simulink model "SCF"  (R2021b)
settings: configuration reference "CommonModelConfiguration" (kept outside this file)
settings Model: Creator=JELIASS5  LastModifiedBy=JELIASS5
settings ConfigSetRef: SourceName=CommonModelConfiguration  SourceLocation=Base Workspace

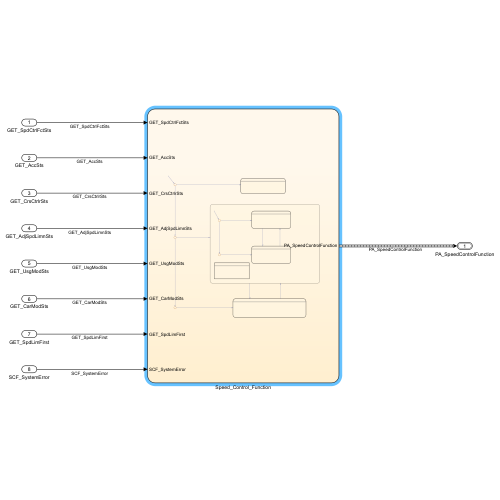
[thumbnail: Simulink's stored preview of the top-level diagram]
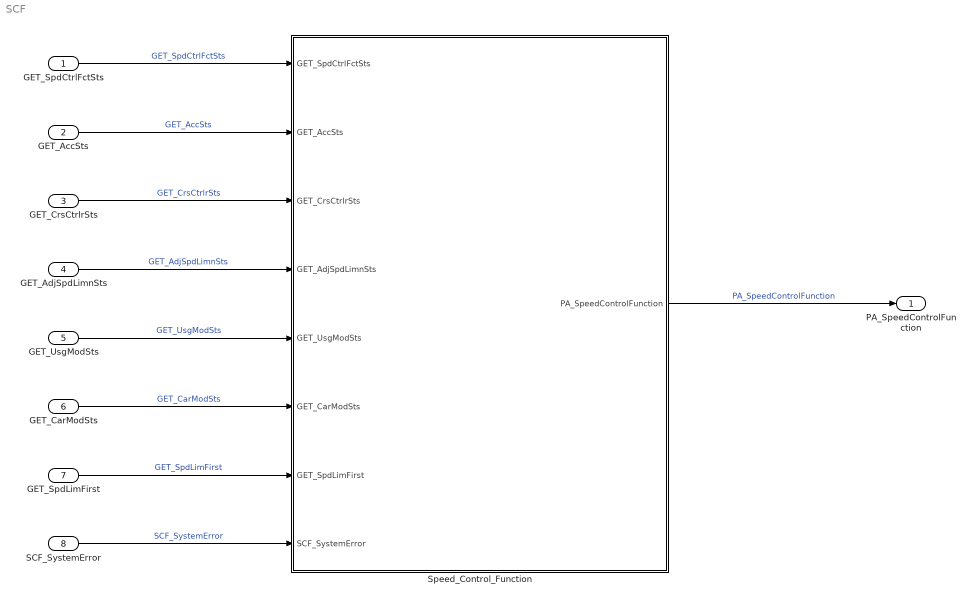
== system SCF ==
  GET_SpdCtrlFctSts : Inport  OutDataTypeStr=Enum: FctStsSpdCtrl
  GET_AccSts : Inport  Port=2  OutDataTypeStr=Enum: AccSts1
  GET_CrsCtrlrSts : Inport  Port=3  OutDataTypeStr=Enum: CrsCtrlrSts1
  GET_AdjSpdLimnSts : Inport  Port=4  OutDataTypeStr=Enum: AdjSpdLimnSts2
  GET_UsgModSts : Inport  Port=5  OutDataTypeStr=Enum: UsgModSts1
  GET_CarModSts : Inport  Port=6  OutDataTypeStr=Enum: CarModSts1
  GET_SpdLimFirst : Inport  Port=7  OutDataTypeStr=SpdLimVal1
  SCF_SystemError : Inport  Port=8  OutDataTypeStr=boolean
  Speed_Control_Function : Stateflow chart  TreatAsAtomicUnit=on
  PA_SpeedControlFunction : Outport  OutDataTypeStr=Bus: PA_StatusAnduIntAndOffOnValue
  wires:
  GET_SpdCtrlFctSts/1 -> Speed_Control_Function/1(GET_SpdCtrlFctSts)  "GET_SpdCtrlFctSts"
  GET_AccSts/1 -> Speed_Control_Function/2(GET_AccSts)  "GET_AccSts"
  GET_CrsCtrlrSts/1 -> Speed_Control_Function/3(GET_CrsCtrlrSts)  "GET_CrsCtrlrSts"
  GET_AdjSpdLimnSts/1 -> Speed_Control_Function/4(GET_AdjSpdLimnSts)  "GET_AdjSpdLimnSts"
  GET_UsgModSts/1 -> Speed_Control_Function/5(GET_UsgModSts)  "GET_UsgModSts"
  GET_CarModSts/1 -> Speed_Control_Function/6(GET_CarModSts)  "GET_CarModSts"
  Speed_Control_Function/1(PA_SpeedControlFunction) -> PA_SpeedControlFunction/1  "PA_SpeedControlFunction"
  GET_SpdLimFirst/1 -> Speed_Control_Function/7(GET_SpdLimFirst)  "GET_SpdLimFirst"
  SCF_SystemError/1 -> Speed_Control_Function/8(SCF_SystemError)  "SCF_SystemError"

== stateflow chart SCF/Speed_Control_Function ==
  state CARCONFIG_INVALID
    en, du:
    PA_SpeedControlFunction.Status = E_CommonStatus.NotPresent;
    PA_SpeedControlFunction.Value = E_OffOn.Off;
    PA_SpeedControlFunction.Data = 0;
  state SYSTEM_OK
    state NOT_ACTIVE
      en, du:
      PA_SpeedControlFunction.Status = E_CommonStatus.Disabled;
      PA_SpeedControlFunction.Value = E_OffOn.Off;
      PA_SpeedControlFunction.Data = 0;
    state ACTIVE
      en, du: PA_SpeedControlFunction.Status = E_CommonStatus.Available;
      state SCF_OFF
        en, du: PA_SpeedControlFunction.Value = E_OffOn.Off;
        PA_SpeedControlFunction.Data = 0;
      state SCF_ON
        en, du: PA_SpeedControlFunction.Value = E_OffOn.On;
        PA_SpeedControlFunction.Data = GET_SpdLimFirst;
      (default) -> SCF_OFF
      SCF_OFF -> SCF_ON : % Speed Control Function is activated
          | [GET_SpdCtrlFctSts == FctStsSpdCtrl.FctStsSpdCtrl_Active ||...
          | GET_SpdCtrlFctSts == FctStsSpdCtrl.FctStsSpdCtrl_Inactive ||...
          | GET_SpdCtrlFctSts == FctStsSpdCtrl.FctStsSpdCtrl_ActiveControlling]
      SCF_ON -> SCF_OFF : %Speed Control Function is deactivated
          | [GET_SpdCtrlFctSts ~= FctStsSpdCtrl.FctStsSpdCtrl_Active &&...
          | GET_SpdCtrlFctSts ~= FctStsSpdCtrl.FctStsSpdCtrl_Inactive &&...
          | GET_SpdCtrlFctSts ~= FctStsSpdCtrl.FctStsSpdCtrl_ActiveControlling]
    state isActive = activationCheck [function]
      (default) -> (junction 32)
      (junction 32) -> (junction 33) [order 1] : [GET_UsgModSts == UsgModSts1.UsgModSts1_UsgModDrvg &&...
          | GET_CarModSts == CarModSts1.CarModSts1_CarModNorm &&...
          | (GET_AccSts == AccSts1.AccSts1_Off || GET_AccSts == AccSts1.AccSts1_Stb) &&...
          | GET_CrsCtrlrSts ~= CrsCtrlrSts1.CrsCtrlrSts1_Actv &&...
          | GET_AdjSpdLimnSts ~= AdjSpdLimnSts2.AdjSpdLimnSts2_Actv &&...
          | GET_AdjSpdLimnSts ~= AdjSpdLimnSts2.AdjSpdLimnSts2_Ovrd]
      (junction 32) -> (junction 34) [order 2] : {isActive = false;}
      (junction 33) -> (junction 35) : {isActive = true;}
      (junction 35) -> (junction 34)
      (junction 34) -> (junction 36)
    (default) -> (junction 22)
    (junction 22) -> NOT_ACTIVE [order 1] : [~activationCheck()]
    (junction 22) -> (junction 25) [order 2]
    NOT_ACTIVE -> ACTIVE : [activationCheck()]
    ACTIVE -> NOT_ACTIVE : [~activationCheck()]
    (junction 25) -> ACTIVE
  state SYSTEM_ERROR
    en, du: PA_SpeedControlFunction.Status = E_CommonStatus.SystemError;
    SYSTEM_ERROR -> (junction 63) [order 1]
    (junction 63) -> (junction 66) [order 1] : %ACC and CC are not active
        | [(GET_AccSts == AccSts1.AccSts1_Off || GET_AccSts == AccSts1.AccSts1_Stb) &&...
        | (GET_CrsCtrlrSts == CrsCtrlrSts1.CrsCtrlrSts1_Off || GET_CrsCtrlrSts == CrsCtrlrSts1.CrsCtrlrSts1_Stb)]
    (junction 63) -> (junction 65) [order 2] : %ACC or CC active and return to user SetSpeed
        | {PA_SpeedControlFunction.Value = E_OffOn.Off;}
    (junction 66) -> (junction 69) : %SetSpeed set to maximum value
        | {PA_SpeedControlFunction.Data = 255;
        | PA_SpeedControlFunction.Value = E_OffOn.On;}
    (junction 69) -> (junction 65)
    (junction 65) -> (junction 72)
  (default) -> (junction 10)
  (junction 10) -> CARCONFIG_INVALID [order 2]
  (junction 10) -> (junction 12) [order 1] : %with SCF
      | [cc_param_251 == 2 || 4]
  (junction 12) -> SYSTEM_OK [order 1] : [SCF_SystemError == false]
  (junction 12) -> (junction 59) [order 2]
  SYSTEM_OK -> SYSTEM_ERROR : [SCF_SystemError == true]
  SYSTEM_ERROR -> SYSTEM_OK [order 1] : [SCF_SystemError == false]
  (junction 59) -> SYSTEM_ERROR
  data: isActive function_output; GET_SpdCtrlFctSts input Enum: FctStsSpdCtrl; GET_AccSts input Enum: AccSts1; GET_CrsCtrlrSts input Enum: CrsCtrlrSts1; GET_AdjSpdLimnSts input Enum: AdjSpdLimnSts2; GET_UsgModSts input Enum: UsgModSts1; GET_CarModSts input Enum: CarModSts1; PA_SpeedControlFunction output Bus: PA_StatusAnduIntAndOffOnValue; cc_param_251 parameter uint8; GET_SpdLimFirst input SpdLimVal1; SCF_SystemError input boolean
